simulink model "Noa_Nofusion"  (R2020b)
settings: Solver=FixedStepDiscrete  StartTime=0.0  StopTime=Inf  FixedStep=0.01  RelTol=1e-3
PostLoadFcn:
  | if any(exist('dsrtsu_mdlpostloadfcn', 'file') ~= 0), dsrtsu_mdlpostloadfcn('Execute', bdroot); end
InitFcn:
  | , if any(exist('rtifpga_mdlclblib', 'file') ~= 0), rtifpga_mdlclblib('Init', bdroot); end,
  | , if any(exist('dsmpb_private', 'file') ~= 0), dsmpb_private('dsmpb_mdlclblib', 'Init', bdroot); end,
undefined symbols (not defined in the file or in its folder): ACC_TimeGap_DecSetSwt, ACC_TimeGap_IncSetSwt, AccelPedalPosn, AccelPedalPosnVldty, AccelPedlPosnDiagc, AccPedalOverride, ACU_ShiftInProgress, ADAS_Posn_CurLane, AESSwtReq, ALC_SwtReq, BrkPedalSts, CC_ACC_CANCEL_OFFSwt, CC_ACC_CRUISE_OFFSwt, CC_ACC_DecSetSpd_SetSwt, CC_ACC_IncSetSpd_ResuSwt, CC_ACCSwtErr, CharSpd_ms, CSA_NODE, CURRENT_GEAR, CurrentGearValid, DiscIntNeverNeededParam, DrvDoorSts, DrvSBR, DrvTrqReqOvld, ECMACCInterface, ECMRespACC, ELKSwtReq, EngLimpHomeSts, EngSpd, EngState, EngState_PHEV, EngTrqMaxActSpd, EngTrqMinAct, EPS_DrvInpTrqVal_HighReslolution, EPS_FailSts, EPS_LKATorqOvrlDlvd, EPS_LKATorqOvrlDlvdVld, EPS_LKATrqOvlDlvdSts, EPS_SteerMod, EPS_TrqSnsrSts, EQ4_APPINFO, EQ4_LA_ELEM, EQ4_LA_HDR, EQ4_LAP_ELEM, EQ4_LAP_HDR, EQ4_LH_ELEM, EQ4_LH_HDR, EQ4_LRE_ELEM, EQ4_LRE_HDR, ESS_PedSwtReq, ESS_VehSwtReq, FFogLmpSts_F_Pbox, FLWheelDriveDirection, FLWheelSpd, FrntWiprSwtSts, FrntWshrSwtSts, FRWheelDriveDirection, FRWheelSpd, HazardLmpSwtSts, HCU_AccelPedalPosn_Diag ... (+151)
libraries: simulink x144, dsmpblib x33, canfdmsglib x10
(part 9 of 20)

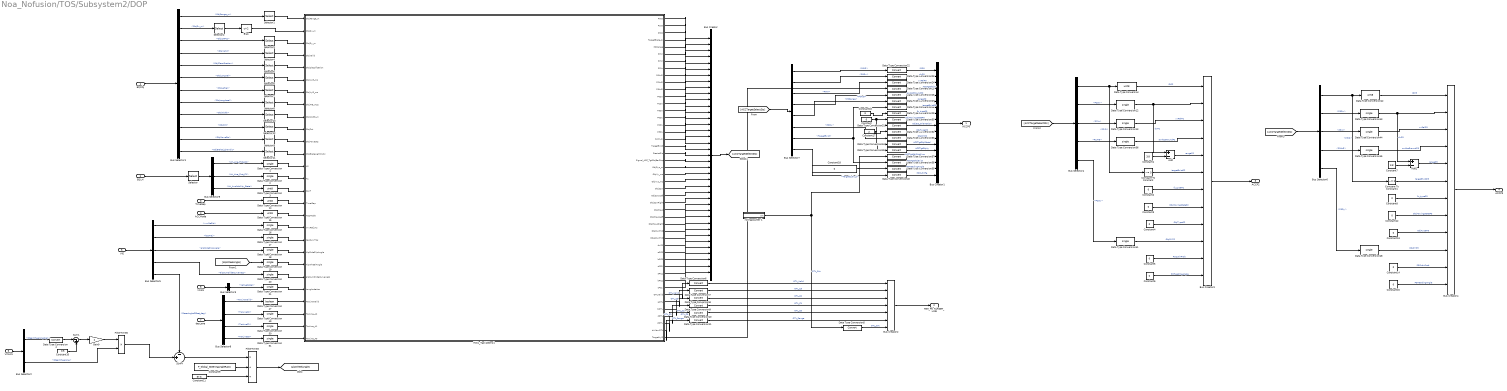
== system Noa_Nofusion/TOS/Subsystem2/DOP ==
  EQObj : Inport
  EQLH : Inport  Port=2
  TimeGap : Inport  Port=3
  ACCMode : Inport  Port=4
  VIE : Inport  Port=5
  VCAN : Inport  Port=6
  desLane : Inport  Port=7
  Add : Sum  Inputs=+-
  Add1 : Sum  Inputs=+-
  Bias : Bias  Bias=2
  Bus Creator : BusCreator  Inputs=39
  Bus Creator1 : BusCreator  Inputs=18  OutDataTypeStr=Bus: TOS_ACCP0_BUS  NonVirtualBus=on
  Bus Creator2 : BusCreator  Inputs=7  OutDataTypeStr=Bus: TOS_P0_TARGET_LINE_BUS  NonVirtualBus=on
  Bus Creator3 : BusCreator  Inputs=12  OutDataTypeStr=Bus: TOS_ACCP2_BUS  NonVirtualBus=on
  Bus Creator4 : BusCreator  Inputs=12  OutDataTypeStr=Bus: TOS_ACCP3_BUS  NonVirtualBus=on
  Bus Selector4 : BusSelector  OutputSignals=P2ID,P2Dx,P2Vr,P2ArG,P2Dy
  Bus Selector6 : BusSelector  OutputSignals=P3ID,P3Dx,P3Vr,P3ArG,P3Dy
  Bus Selector7 : BusSelector  OutputSignals=P0ID,P0Dx,P0Vr,P0ArG,P0Range,P0Dy,TargetExist,TargetCutIn_b
  Bus Selector9 : BusSelector  OutputSignals=LH_Line_First_C2,LH_Line_First_C1,LH_Availability_State
  Bus Selector1 : BusSelector  OutputSignals=ObjRange_m,ObjDx_m,ObjLatPos,ObjValid,ObjClassification,ObjLongVel,ObjLatVel,ObjLongAccel,ObjWidth,ObjCnt,ObjMoveSts,ObjBrakeLightIndic
  Bus Selector2 : BusSelector  OutputSignals=CSA_NODE.CSA2_MSG.SteerWheelAngSign,CSA_NODE.CSA2_MSG.SteerWheelAng
  Bus Selector3 : BusSelector  OutputSignals=ABM_NODE.ABM2_MSG.VehLgtAccel
  Bus Selector5 : BusSelector  OutputSignals=vxvRefMs,kapTraj,alpSideSlipAngle,alpSumSlideCurveness,SteerAngleOffset_deg
  Bus Selector8 : BusSelector  OutputSignals=TarLineValid,TarLineC2,TarLineC1,TarLineC0
  Compare To Constant : simulink/Logic and Bit Operations/Compare To Constant  relop=~=  const=0  OutDataTypeStr=boolean
  Compare To Constant1 : simulink/Logic and Bit Operations/Compare To Constant  relop=~=  const=0  OutDataTypeStr=boolean
  Constant : Constant  Value=0
  Constant1 : Constant  Value=3.8  OutDataTypeStr=single
  Constant10 : Constant  Value=0.5  OutDataTypeStr=single
  Constant11 : Constant  Value=57.3  OutDataTypeStr=single
  Constant{2..4,8,12..13} (6 alike) : Constant  Value=0  OutDataTypeStr=uint8
  Constant{5..6,14..15} (4 alike) : Constant  Value=0  OutDataTypeStr=single
  Constant16 : Constant  Value=3
  Constant17 : Constant  Value=2
  Constant18 : Constant  Value=0
  Constant7 : Constant  Value=3.8  OutDataTypeStr=single
  Constant9 : Constant  Value=P_Global_SteeringAngleRatio
  Data Type Conversion{,3,14..15,42} (5 alike) : DataTypeConversion  OutDataTypeStr=uint8
  Data Type Conversion{1..2,12..13,16..21,36,41,43..45,48..51} (19 alike) : DataTypeConversion  OutDataTypeStr=single
  Data Type Conversion{4..11,22..35,37..40} (26 alike) : DataTypeConversion
  Data Type Conversion47 : DataTypeConversion  OutDataTypeStr=boolean
  FilterTime3 : Product  Inputs=*//  RndMeth=Zero
  FilterTime6 : Product  Inputs=**  RndMeth=Zero
  Gain9 : Gain  Gain=2
  HWA_Task100ms1 : Subsystem
  Selector : Selector  InputPortWidth=2  IndexOptions=Index vector (dialog)  Indices=1  OutputSizes=1
  Selector{1..12} (12 alike) : Selector  InputPortWidth=20  IndexOptions=Index vector (dialog)  Indices=[1:15]  OutputSizes=1
  Sum1 : Sum  Inputs=|-+
  Sum4 : Sum  Inputs=-+|
  VCAN1 : InportShadow  Port=6
  rollingcounter 1 : Subsystem
  ACCP0 : Outport  OutDataTypeStr=Bus: TOS_ACCP0_BUS
  TEM_P0_TARGET_LINE : Outport  Port=2  OutDataTypeStr=Bus: TOS_P0_TARGET_LINE_BUS  PortDimensions=1  BusOutputAsStruct=on
  ACCP2 : Outport  Port=3  OutDataTypeStr=Bus: TOS_ACCP2_BUS
  ACCP3 : Outport  Port=4  OutDataTypeStr=Bus: TOS_ACCP3_BUS
  wires:
  EQLH/1 -> Selector/1
  EQObj/1 -> Bus Selector1/1
  Bus Selector8/4 -> Data Type Conversion51/1  "<TarLineC0>"
  Data Type Conversion51/1 -> HWA_Task100ms1/27(TarLine_A0)
  Constant18/1 -> Data Type Conversion39/1
  HWA_Task100ms1/46(TargetVyG) -> Data Type Conversion25/1
  Constant17/1 -> Data Type Conversion32/1
  Constant16/1 -> Data Type Conversion29/1
  Selector2/1 -> Bias/1
  [ACCTargetSelectSts] -> Bus Selector6/1
  Bus Selector6/1 -> Compare To Constant1/1, Data Type Conversion42/1  "<P3ID>"
  Data Type Conversion42/1 -> Bus Creator4/1  "IDP3"
  Bus Selector6/2 -> Data Type Conversion43/1  "<P3Dx>"
  Data Type Conversion43/1 -> Add1/1, Bus Creator4/2  "dxP3"
  Bus Selector6/3 -> Data Type Conversion44/1  "<P3Vr>"
  Data Type Conversion44/1 -> Bus Creator4/3  "vxRelP3"
  Bus Selector6/4 -> Data Type Conversion45/1  "<P3ArG>"
  Data Type Conversion45/1 -> Bus Creator4/4  "axAbsGroundP3"
  Add1/1 -> Bus Creator4/5  "rangeP3"
  Constant7/1 -> Add1/2
  Compare To Constant1/1 -> Bus Creator4/6  "targetExistP3"
  Constant8/1 -> Bus Creator4/7  "fu_typeP3"
  Constant12/1 -> Bus Creator4/8  "ObjMovingStateP3"
  Constant13/1 -> Bus Creator4/9  "ObjTypeP3"
  Bus Selector6/5 -> Data Type Conversion48/1  "<P3Dy>"
  Data Type Conversion48/1 -> Bus Creator4/10  "ObjDYP3"
  Constant14/1 -> Bus Creator4/11  "P3CutinProb"
  Constant15/1 -> Bus Creator4/12  "P3HeadingAngle"
  Bus Creator4/1 -> ACCP3/1
  Bus Creator3/1 -> ACCP2/1
  Constant6/1 -> Bus Creator3/12  "P2HeadingAngle"
  Constant5/1 -> Bus Creator3/11  "P2CutinProb"
  Data Type Conversion41/1 -> Bus Creator3/10  "ObjDYP2"
  Bus Selector4/5 -> Data Type Conversion41/1  "<P2Dy>"
  Constant4/1 -> Bus Creator3/9  "ObjTypeP2"
  Constant3/1 -> Bus Creator3/8  "ObjMovingStateP2"
  Constant2/1 -> Bus Creator3/7  "fu_typeP2"
  Compare To Constant/1 -> Bus Creator3/6  "targetExistP2"
  Constant1/1 -> Add/2
  Add/1 -> Bus Creator3/5  "rangeP2"
  Data Type Conversion36/1 -> Bus Creator3/4  "axAbsGroundP2"
  Bus Selector4/4 -> Data Type Conversion36/1  "<P2ArG>"
  Data Type Conversion13/1 -> Bus Creator3/3  "vxRelP2"
  Bus Selector4/3 -> Data Type Conversion13/1  "<P2Vr>"
  Data Type Conversion12/1 -> Bus Creator3/2, Add/1  "dxP2"
  Bus Selector4/2 -> Data Type Conversion12/1  "<P2Dx>"
  Data Type Conversion/1 -> Bus Creator3/1  "IDP2"
  Bus Selector4/1 -> Data Type Conversion/1, Compare To Constant/1  "<P2ID>"
  [ACCTargetSelectSts] -> Bus Selector4/1
  Selector12/1 -> HWA_Task100ms1/10(ObjCnt)
  Selector11/1 -> HWA_Task100ms1/12(ObjBrakeLightIndic)
  Selector10/1 -> HWA_Task100ms1/9(ObjWidth_m)
  Selector9/1 -> HWA_Task100ms1/11(ObjMoveSts)
  Selector8/1 -> HWA_Task100ms1/8(ObjArG_ms2)
  Selector7/1 -> HWA_Task100ms1/7(ObjVyG_ms)
  Selector6/1 -> HWA_Task100ms1/6(ObjVxG_ms)
  Selector5/1 -> HWA_Task100ms1/5(ObjClassification)
  Selector4/1 -> HWA_Task100ms1/4(ObjValid)
  Selector3/1 -> HWA_Task100ms1/3(ObjDy_m)
  Bias/1 -> HWA_Task100ms1/2(ObjDx_m)
  Selector1/1 -> HWA_Task100ms1/1(ObjRange_m)
  Selector/1 -> Bus Selector9/1
  Data Type Conversion11/1 -> Bus Creator2/6  "OTL_Range"
  Data Type Conversion10/1 -> Bus Creator2/5  "OTL_C0"
  Data Type Conversion9/1 -> Bus Creator2/4  "OTL_C1"
  Data Type Conversion8/1 -> Bus Creator2/3  "OTL_C2"
  Data Type Conversion7/1 -> Bus Creator2/2  "OTL_C3"
  Data Type Conversion6/1 -> Bus Creator2/1  "OTL_Valid"
  Data Type Conversion5/1 -> Bus Creator2/7  "OTL_Cnt"
  Bus Creator2/1 -> TEM_P0_TARGET_LINE/1
  HWA_Task100ms1/42(bOTL) -> Data Type Conversion8/1  "OTL_C2"
  HWA_Task100ms1/41(aOTL) -> Data Type Conversion7/1  "OTL_C3"
  HWA_Task100ms1/40(OTLValid) -> Data Type Conversion6/1  "OTL_Valid"
  HWA_Task100ms1/43(cOTL) -> Data Type Conversion9/1  "OTL_C1"
  rollingcounter 1/1(cnt) -> Data Type Conversion5/1, Data Type Conversion37/1  "OTL_Cnt"
  HWA_Task100ms1/45(dxMaxOTL) -> Data Type Conversion11/1  "OTL_Range"
  HWA_Task100ms1/44(dOTL) -> Data Type Conversion10/1  "OTL_C0"
  Data Type Conversion4/1 -> Sum1/1
  Bus Selector2/2 -> FilterTime6/2  "<SteerWheelAng>"
  Bus Selector2/1 -> Data Type Conversion4/1  "<SteerWheelAngSign>"
  Sum1/1 -> Gain9/1
  Gain9/1 -> FilterTime6/1
  Constant10/1 -> Sum1/2
  VCAN1/1 -> Bus Selector2/1
  Constant9/1 -> FilterTime3/2
  Bus Selector5/5 -> Sum4/1  "<SteerAngleOffset_deg>"
  FilterTime3/1 -> [alpWheelAngle]
  Sum4/1 -> FilterTime3/1
  Constant11/1 -> FilterTime3/3
  FilterTime6/1 -> Sum4/2
  HWA_Task100ms1/34(aPC0) -> Bus Creator/34
  HWA_Task100ms1/38(bPC1) -> Bus Creator/38
  Bus Selector7/1 -> Data Type Conversion22/1  "<P0ID>"
  Data Type Conversion3/1 -> HWA_Task100ms1/15(Conf)
  Data Type Conversion22/1 -> Bus Creator1/1  "IDP0"
  Data Type Conversion27/1 -> Bus Creator1/6  "rangeP0"
  Data Type Conversion1/1 -> HWA_Task100ms1/13(A2)
  HWA_Task100ms1/2(P2ID) -> Bus Creator/2
  Data Type Conversion2/1 -> HWA_Task100ms1/14(A1)
  Data Type Conversion37/1 -> Bus Creator1/15  "ACCTgtObjCntAlive"
  HWA_Task100ms1/1(P0ID) -> Bus Creator/1
  Bus Selector3/1 -> Data Type Conversion21/1  "<VehLgtAccel>"
  Bus Selector1/9 -> Selector10/1  "<ObjWidth>"
  Data Type Conversion19/1 -> HWA_Task100ms1/21(AlpWheelAngle)
  Bus Selector7/3 -> Data Type Conversion24/1  "<P0Vr>"
  Bus Selector9/1 -> Data Type Conversion1/1  "<LH_Line_First_C2>"
  VIE/1 -> Bus Selector5/1
  Bus Creator1/1 -> ACCP0/1
  Data Type Conversion38/1 -> Bus Creator1/16  "ACCTgtObjExist"
  Bus Selector7/6 -> Data Type Conversion33/1  "<P0Dy>"
  Bus Selector7/2 -> Data Type Conversion23/1  "<P0Dx>"
  Data Type Conversion29/1 -> Bus Creator1/8  "fu_typeP0"
  Bus Selector7/8 -> Data Type Conversion40/1  "<TargetCutIn_b>"
  HWA_Task100ms1/32(ObjqDycHist) -> Bus Creator/32
  Data Type Conversion32/1 -> Bus Creator1/11  "ObjTypeP0"
  Data Type Conversion35/1 -> Bus Creator1/14  "ACCTgtObjAy"
  VCAN/1 -> Bus Selector3/1
  Data Type Conversion34/1 -> Bus Creator1/13  "ACCTgtObjObstcl"
  Bus Selector8/1 -> Data Type Conversion47/1  "<TarLineValid>"
  Bus Selector5/1 -> Data Type Conversion16/1  "<vxvRefMs>"
  Data Type Conversion17/1 -> HWA_Task100ms1/19(kapCurvTraj)
  Data Type Conversion28/1 -> Bus Creator1/7  "targetExistP0"
  Bus Selector1/7 -> Selector7/1  "<ObjLatVel>"
  HWA_Task100ms1/8(P3Vr) -> Bus Creator/8
  Bus Selector1/8 -> Selector8/1  "<ObjLongAccel>"
  Data Type Conversion49/1 -> HWA_Task100ms1/25(TarLine_A2)
  ACCMode/1 -> Data Type Conversion15/1
  HWA_Task100ms1/22(ObjDyc_m) -> Bus Creator/22
  Data Type Conversion18/1 -> HWA_Task100ms1/20(AlpSideSlipAngle)
  Data Type Conversion30/1 -> Bus Creator1/9  "ObjMovingStateP0"
  HWA_Task100ms1/11(P3ArG) -> Bus Creator/11
  Data Type Conversion25/1 -> Bus Creator1/4  "ACCTgtObjVy"
  TimeGap/1 -> Data Type Conversion14/1
  Data Type Conversion23/1 -> Bus Creator1/2  "dxP0"
  Data Type Conversion21/1 -> HWA_Task100ms1/23(LongitudeAcc)
  Bus Creator/1 -> [ACCTargetSelectSts]
  HWA_Task100ms1/31(ObjDycHist) -> Bus Creator/31
  Bus Selector1/5 -> Selector5/1  "<ObjClassification>"
  Bus Selector7/5 -> Data Type Conversion27/1  "<P0Range>"
  Bus Selector5/2 -> Data Type Conversion17/1  "<kapTraj>"
  Bus Selector1/3 -> Selector3/1  "<ObjLatPos>"
  Constant/1 -> Data Type Conversion30/1, Data Type Conversion31/1, Data Type Conversion34/1, Data Type Conversion35/1
  Data Type Conversion47/1 -> HWA_Task100ms1/24(TarLineValid)
  HWA_Task100ms1/4(TargetBrake_b) -> Bus Creator/4
  Data Type Conversion14/1 -> HWA_Task100ms1/16(TimeGap)
  HWA_Task100ms1/15(P0Dy) -> Bus Creator/15
  HWA_Task100ms1/33(dxC0) -> Bus Creator/33
  Data Type Conversion39/1 -> Bus Creator1/17  "P0HeadingAngle"
  HWA_Task100ms1/21(Signal_ACC_TgtObjBarDisp) -> Bus Creator/21
  HWA_Task100ms1/24(ObjVyc_ms) -> Bus Creator/24
  HWA_Task100ms1/16(P2Dy) -> Bus Creator/16
  Bus Selector8/3 -> Data Type Conversion50/1  "<TarLineC1>"
  HWA_Task100ms1/30(ObjPlausRight) -> Bus Creator/30
  HWA_Task100ms1/13(P2Dx) -> Bus Creator/13
  Bus Selector1/11 -> Selector9/1  "<ObjMoveSts>"
  HWA_Task100ms1/35(bPC0) -> Bus Creator/35
  Data Type Conversion16/1 -> HWA_Task100ms1/18(VxvRef_ms)
  Bus Selector9/2 -> Data Type Conversion2/1  "<LH_Line_First_C1>"
  HWA_Task100ms1/18(CutIn_b) -> Bus Creator/18
  HWA_Task100ms1/27(ObjSpwRight) -> Bus Creator/27
  [ACCTargetSelectSts] -> Bus Selector7/1
  HWA_Task100ms1/3(P3ID) -> Bus Creator/3
  HWA_Task100ms1/20(DesireDis) -> Bus Creator/20
  Bus Selector7/4 -> Data Type Conversion26/1  "<P0ArG>"
  Data Type Conversion31/1 -> Bus Creator1/10  "Object_Orientation"
  Data Type Conversion50/1 -> HWA_Task100ms1/26(TarLine_A1)
  Bus Selector1/1 -> Selector1/1  "<ObjRange_m>"
  Bus Selector1/6 -> Selector6/1  "<ObjLongVel>"
  Bus Selector1/12 -> Selector11/1  "<ObjBrakeLightIndic>"
  Bus Selector5/3 -> Data Type Conversion18/1  "<alpSideSlipAngle>"
  HWA_Task100ms1/14(P3Dx) -> Bus Creator/14
  Data Type Conversion33/1 -> Bus Creator1/12  "ObjDYP0"
  Bus Selector5/4 -> Data Type Conversion20/1  "<alpSumSlideCurveness>"
  HWA_Task100ms1/9(P0ArG) -> Bus Creator/9
  HWA_Task100ms1/36(cPC0) -> Bus Creator/36
  HWA_Task100ms1/39(cPC1) -> Bus Creator/39
  HWA_Task100ms1/12(P0Dx) -> Bus Creator/12
  HWA_Task100ms1/17(P3Dy) -> Bus Creator/17
  HWA_Task100ms1/19(TargetExist) -> Bus Creator/19
  Bus Selector1/10 -> Selector12/1  "<ObjCnt>"
  HWA_Task100ms1/10(P2ArG) -> Bus Creator/10
  HWA_Task100ms1/26(ObjSpwLeft) -> Bus Creator/26
  HWA_Task100ms1/37(aPC1) -> Bus Creator/37
  HWA_Task100ms1/5(P0Range) -> Bus Creator/5
  Data Type Conversion26/1 -> Bus Creator1/5  "axAbsGroundP0"
  Bus Selector1/2 -> Selector2/1  "<ObjDx_m>"
  HWA_Task100ms1/28(ObjPlaus) -> Bus Creator/28
  Data Type Conversion24/1 -> Bus Creator1/3  "vxRelP0"
  Bus Selector8/2 -> Data Type Conversion49/1  "<TarLineC2>"
  Bus Selector1/4 -> Selector4/1  "<ObjValid>"
  HWA_Task100ms1/7(P2Vr) -> Bus Creator/7
  HWA_Task100ms1/29(ObjPlausLeft) -> Bus Creator/29
  Data Type Conversion40/1 -> Bus Creator1/18  "P0CutInflg"
  desLane/1 -> Bus Selector8/1
  Bus Selector9/3 -> Data Type Conversion3/1  "<LH_Availability_State>"
  [alpWheelAngle] -> Data Type Conversion19/1
  HWA_Task100ms1/25(ObjSpw) -> Bus Creator/25
  HWA_Task100ms1/6(P0Vr) -> Bus Creator/6
  Bus Selector7/7 -> Data Type Conversion38/1, Data Type Conversion28/1  "<TargetExist>"
  Data Type Conversion15/1 -> HWA_Task100ms1/17(ACCMode)
  HWA_Task100ms1/23(ObjVy_ms) -> Bus Creator/23
  Data Type Conversion20/1 -> HWA_Task100ms1/22(alpSumSlideCurveness)

== system Noa_Nofusion/TOS/Subsystem2/ObjMatrixTransit ==
  EQ4_OBJ : Inport
  Bus Creator : BusCreator  Inputs=14
  Bus Selector4 : BusSelector  OutputSignals=EQ4_OBJ_HDR.OBJ_Sync_ID,EQ4_OBJ_HDR.OBJ_VRU_Count,EQ4_OBJ_HDR.OBJ_VD_Count,EQ4_OBJ_HDR.OBJ_General_OBJ_Count,EQ4_OBJ_HDR.OBJ_Animal_Count,EQ4_OBJ_ELEM
  Data Type Conversion : DataTypeConversion
  IFV2FrontBumper : Constant  Value=1.7  OutDataTypeStr=single
  IFV2RearAxis : Constant  Value=2.1  OutDataTypeStr=single
  Subsystem : Subsystem
  Sum : Sum  Inputs=++++
  Sum1 : Sum  Inputs=|-+
  Sum5 : Sum  Inputs=++|
  Terminator1 : Terminator
  VisObj : Outport
  wires:
  Subsystem/13(P) -> Terminator1/1
  EQ4_OBJ/1 -> Bus Selector4/1
  Bus Selector4/5 -> Sum/4  "<OBJ_Animal_Count>"
  Bus Selector4/1 -> Data Type Conversion/1  "<OBJ_Sync_ID>"
  Bus Selector4/2 -> Sum/1  "<OBJ_VRU_Count>"
  Bus Selector4/3 -> Sum/2  "<OBJ_VD_Count>"
  Bus Selector4/4 -> Sum/3  "<OBJ_General_OBJ_Count>"
  Sum/1 -> Subsystem/1(Count)
  Bus Selector4/6 -> Subsystem/2(<EQ4_OBJ_ELEM>)  "<EQ4_OBJ_ELEM>"
  Subsystem/1(ObjID) -> Bus Creator/2  "ObjID"
  Bus Creator/1 -> VisObj/1  "ObjSts"
  IFV2FrontBumper/1 -> Sum1/1
  Data Type Conversion/1 -> Bus Creator/1  "Cnt"
  IFV2RearAxis/1 -> Sum5/2
  Sum5/1 -> Bus Creator/14  "ObjDx_m"
  Subsystem/11(ObjMoveSts) -> Bus Creator/12  "ObjMoveSts"
  Sum1/1 -> Bus Creator/13  "ObjRange_m"
  Subsystem/10(ObjCnt) -> Bus Creator/11  "ObjCnt"
  Subsystem/8(ObjLongVel) -> Bus Creator/9  "ObjLongVel"
  Subsystem/12(ObjLongPos) -> Sum1/2, Sum5/1
  Subsystem/9(ObjWidth) -> Bus Creator/10  "ObjWidth"
  Subsystem/3(ObjBrakeLightIndic) -> Bus Creator/4  "ObjBrakeLightIndic"
  Subsystem/5(ObjLatPos) -> Bus Creator/6  "ObjLatPos"
  Subsystem/7(ObjLongAccel) -> Bus Creator/8  "ObjLongAccel"
  Subsystem/2(ObjValid) -> Bus Creator/3  "ObjValid"
  Subsystem/4(ObjClassification) -> Bus Creator/5  "ObjClassification"
  Subsystem/6(ObjLatVel) -> Bus Creator/7  "ObjLatVel"

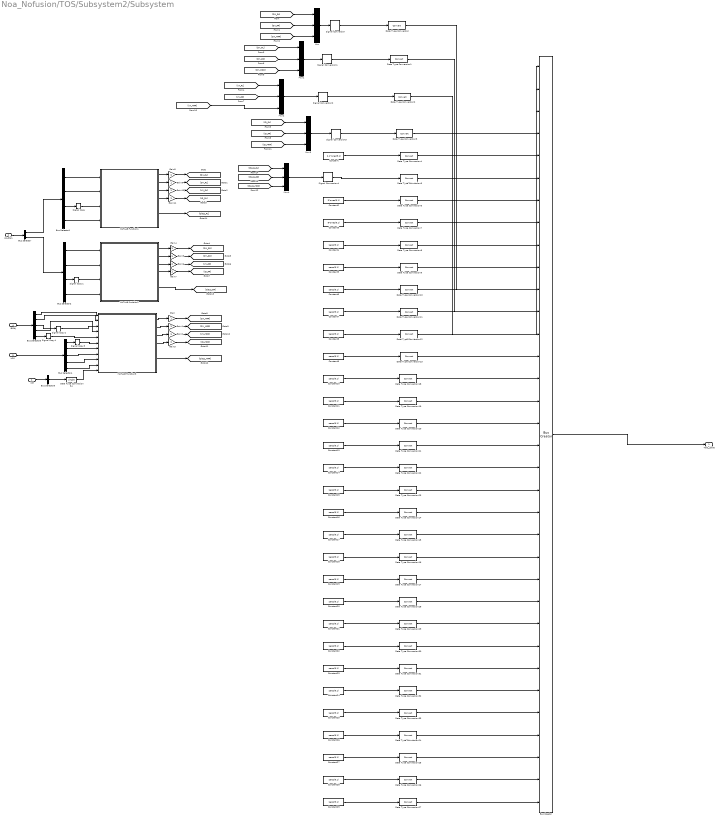
== system Noa_Nofusion/TOS/Subsystem2/Subsystem ==
  VIE : Inport
  LC_Obj1 : Inport  Port=2
  LSM : Inport  Port=3
  IEObj : Inport  Port=4
  Bus Creator : BusCreator  Inputs=34  OutDataTypeStr=Bus: TOS_LCKIE_BUS  NonVirtualBus=on
  Bus Selector : BusSelector  OutputSignals=RL,RR
  Bus Selector1 : BusSelector  OutputSignals=ObjID,ObjDy,ObjDx,ObjVx
  Bus Selector2 : BusSelector  OutputSignals=ObjID,ObjDy,ObjDx,ObjVx
  Bus Selector3 : BusSelector  OutputSignals=ObjID,ObjLatPos,ObjDx_m,ObjLongVel,ObjClass
  Bus Selector4 : BusSelector  OutputSignals=LSM_LCK.LCKLineValid,LSM_LCK.LCKLineC0,LSM_LCK.LCKLineC1,LSM_LCK.LCKLineC2,LSM_LCK.LCKLineC3
  Bus Selector5 : BusSelector  OutputSignals=vxvRefMs
  Constant : Constant  Value=2.1*ones(9,1)  OutDataTypeStr=single
  Constant{4..29} (26 alike) : Constant  Value=zeros(9,1)  OutDataTypeStr=single
  Constant2 : Constant  Value=3*ones(9,1)  OutDataTypeStr=uint8
  Constant3 : Constant  Value=8*ones(9,1)  OutDataTypeStr=single
  Data Type Conversion{,1..33} (34 alike) : DataTypeConversion
  Data Type Conversion34 : DataTypeConversion  OutDataTypeStr=single
  Gain{,1..11} (12 alike) : Gain
  MATLAB Function1 : MATLAB Function  TreatAsAtomicUnit=on
  MATLAB Function2 : MATLAB Function  TreatAsAtomicUnit=on
  MATLAB Function3 : MATLAB Function  TreatAsAtomicUnit=on
  Mux{,1..4} (5 alike) : Mux  Inputs=3
  Signal Conversion{,1..4} (5 alike) : SignalConversion  OverrideOpt=off
  Signal Copy{,1..4} (5 alike) : SignalConversion  OverrideOpt=off
  TOS_LCKIE : Outport  OutDataTypeStr=Bus: TOS_LCKIE_BUS
  wires:
  Bus Selector2/2 -> MATLAB Function2/2(ObjDy)  "<ObjDy>"
  Bus Selector/2 -> Bus Selector2/1  "<RR>"
  LC_Obj1/1 -> Bus Selector/1
  Bus Selector1/3 -> Signal Copy/1  "<ObjDx>"
  Bus Selector1/2 -> MATLAB Function1/2(ObjDy)  "<ObjDy>"
  Bus Selector1/4 -> MATLAB Function1/4(ObjVx)  "<ObjVx>"
  Bus Selector4/3 -> MATLAB Function3/8(C1)  "<LCKLineC1>"
  Bus Selector2/1 -> MATLAB Function2/1(ObjID)  "<ObjID>"
  Bus Selector1/1 -> MATLAB Function1/1(ObjID)  "<ObjID>"
  Bus Selector2/3 -> Signal Copy1/1  "<ObjDx>"
  Bus Selector2/4 -> MATLAB Function2/4(ObjVx)  "<ObjVx>"
  Bus Selector3/4 -> MATLAB Function3/4(ObjVx)  "<ObjLongVel>"
  Bus Selector3/3 -> Signal Copy2/1  "<ObjDx_m>"
  Bus Selector4/2 -> MATLAB Function3/7(C0)  "<LCKLineC0>"
  Bus Selector3/2 -> MATLAB Function3/2(ObjDy)  "<ObjLatPos>"
  Bus Selector3/1 -> MATLAB Function3/1(ObjID)  "<ObjID>"
  LSM/1 -> Bus Selector4/1
  Bus Selector/1 -> Bus Selector1/1  "<RL>"
  Bus Selector4/1 -> Signal Copy3/1  "<LCKLineValid>"
  Bus Selector4/5 -> MATLAB Function3/10(C3)  "<LCKLineC3>"
  Bus Selector4/4 -> MATLAB Function3/9(C2)  "<LCKLineC2>"
  IEObj/1 -> Bus Selector3/1
  MATLAB Function1/1(Dx) -> Gain8/1
  MATLAB Function1/2(Dy) -> Gain9/1
  MATLAB Function1/3(Vx) -> Gain10/1
  MATLAB Function1/4(ID) -> Gain11/1
  MATLAB Function2/1(Dx) -> Gain4/1
  MATLAB Function2/2(Dy) -> Gain5/1
  MATLAB Function2/3(Vx) -> Gain6/1
  MATLAB Function2/4(ID) -> Gain7/1
  MATLAB Function3/1(Dx) -> Gain/1
  MATLAB Function3/2(Dy) -> Gain1/1
  MATLAB Function3/3(Vx) -> Gain2/1
  MATLAB Function3/4(ID) -> Gain3/1
  [DX_RL] -> Mux/1
  [DX_RR] -> Mux/2
  [DX_MRR] -> Mux/3
  [DY_RR] -> Mux1/2
  [DY_RL] -> Mux1/1
  [DY_MRR] -> Mux1/3
  [VX_RL] -> Mux2/1
  [VX_RR] -> Mux2/2
  [ID_RL] -> Mux3/1
  [ID_RR] -> Mux3/2
  [ID_MRR] -> Mux3/3
  Mux/1 -> Signal Conversion/1
  Mux1/1 -> Signal Conversion1/1
  Mux2/1 -> Signal Conversion2/1
  Mux3/1 -> Signal Conversion3/1
  Constant/1 -> Data Type Conversion4/1  "Object_Width"
  Mux4/1 -> Signal Conversion4/1  "Object_Type"
  Constant2/1 -> Data Type Conversion6/1  "Object_Fus_Type"
  Bus Creator/1 -> TOS_LCKIE/1
  Constant3/1 -> Data Type Conversion7/1  "Object_Length"
  Constant4/1 -> Data Type Conversion8/1  "Object_Hight"
  Constant5/1 -> Data Type Conversion9/1  "Object_HeadingAngle"
  Constant6/1 -> Data Type Conversion10/1  "Object_YawAngle"
  Constant7/1 -> Data Type Conversion11/1  "Object_MovingState"
  Constant8/1 -> Data Type Conversion12/1  "Object_Orientation"
  Constant9/1 -> Data Type Conversion13/1  "Object_VY"
  Constant10/1 -> Data Type Conversion18/1  "Object_Std_AX"
  Constant11/1 -> Data Type Conversion19/1  "Object_Std_AY"
  Constant12/1 -> Data Type Conversion20/1  "Object_Std_DX"
  Constant13/1 -> Data Type Conversion21/1  "Object_Std_DY"
  Constant14/1 -> Data Type Conversion22/1  "Object_Std_VX"
  Constant15/1 -> Data Type Conversion23/1  "Object_Std_VY"
  Constant16/1 -> Data Type Conversion14/1  "Object_AX"
  Constant17/1 -> Data Type Conversion15/1  "Object_AY"
  Constant18/1 -> Data Type Conversion16/1  "Object_Std_Length"
  Constant19/1 -> Data Type Conversion17/1  "Object_Std_Width"
  Constant20/1 -> Data Type Conversion28/1  "Object_Std_HeadingAngle"
  Constant21/1 -> Data Type Conversion29/1  "Object_Type_Prob"
  Constant22/1 -> Data Type Conversion30/1  "Object_ExistProb"
  Constant23/1 -> Data Type Conversion31/1  "Object_ObstacleProb"
  Constant24/1 -> Data Type Conversion32/1  "Object_Age"
  Constant25/1 -> Data Type Conversion33/1  "cutIn"
  Constant26/1 -> Data Type Conversion24/1  "CurrentLane_Prob"
  Constant27/1 -> Data Type Conversion25/1  "LeftLane_Prob"
  Constant28/1 -> Data Type Conversion26/1  "RightLane_Prob"
  Constant29/1 -> Data Type Conversion27/1  "ObjectIn_Lane"
  Data Type Conversion/1 -> Bus Creator/11  "Object_DX"
  Data Type Conversion1/1 -> Bus Creator/12  "Object_DY"
  Data Type Conversion2/1 -> Bus Creator/13  "Object_VX"
  Data Type Conversion3/1 -> Bus Creator/2  "Object_ID"
  Data Type Conversion4/1 -> Bus Creator/5  "Object_Width"
  Data Type Conversion5/1 -> Bus Creator/3  "Object_Type"
  Data Type Conversion6/1 -> Bus Creator/1  "Object_Fus_Type"
  Data Type Conversion7/1 -> Bus Creator/4  "Object_Length"
  Data Type Conversion8/1 -> Bus Creator/6  "Object_Hight"
  Data Type Conversion11/1 -> Bus Creator/9  "Object_MovingState"
  Data Type Conversion9/1 -> Bus Creator/7  "Object_HeadingAngle"
  Data Type Conversion10/1 -> Bus Creator/8  "Object_YawAngle"
  Data Type Conversion12/1 -> Bus Creator/10  "Object_Orientation"
  Data Type Conversion13/1 -> Bus Creator/14  "Object_VY"
  Data Type Conversion15/1 -> Bus Creator/22  "Object_AY"
  Data Type Conversion17/1 -> Bus Creator/24  "Object_Std_Width"
  Data Type Conversion18/1 -> Bus Creator/15  "Object_Std_AX"
  Data Type Conversion20/1 -> Bus Creator/17  "Object_Std_DX"
  Data Type Conversion19/1 -> Bus Creator/16  "Object_Std_AY"
  Data Type Conversion22/1 -> Bus Creator/19  "Object_Std_VX"
  Data Type Conversion21/1 -> Bus Creator/18  "Object_Std_DY"
  Data Type Conversion23/1 -> Bus Creator/20  "Object_Std_VY"
  Data Type Conversion24/1 -> Bus Creator/31  "CurrentLane_Prob"
  Data Type Conversion26/1 -> Bus Creator/33  "RightLane_Prob"
  Data Type Conversion25/1 -> Bus Creator/32  "LeftLane_Prob"
  Data Type Conversion29/1 -> Bus Creator/26  "Object_Type_Prob"
  Data Type Conversion30/1 -> Bus Creator/27  "Object_ExistProb"
  Data Type Conversion33/1 -> Bus Creator/30  "cutIn"
  Data Type Conversion32/1 -> Bus Creator/29  "Object_Age"
  Data Type Conversion31/1 -> Bus Creator/28  "Object_ObstacleProb"
  Data Type Conversion28/1 -> Bus Creator/25  "Object_Std_HeadingAngle"
  Data Type Conversion27/1 -> Bus Creator/34  "ObjectIn_Lane"
  Data Type Conversion14/1 -> Bus Creator/21  "Object_AX"
  Data Type Conversion16/1 -> Bus Creator/23  "Object_Std_Length"
  Signal Copy/1 -> MATLAB Function1/3(ObjDx)
  Signal Copy1/1 -> MATLAB Function2/3(ObjDx)
  Signal Copy2/1 -> MATLAB Function3/3(ObjDx)  "EQ4_DX"
  Signal Copy3/1 -> MATLAB Function3/6(L_Valid)
  Signal Conversion/1 -> Data Type Conversion/1  "LCKIE_DX"
  Signal Conversion1/1 -> Data Type Conversion1/1  "LCKIE_DY"
  Signal Conversion2/1 -> Data Type Conversion2/1  "LCKIE_VX"
  Signal Conversion3/1 -> Data Type Conversion3/1  "LCKIE_ID"
  Gain/1 -> [DX_MRR]
  Gain1/1 -> [DY_MRR]
  Gain2/1 -> [VX_MRR]
  Gain3/1 -> [ID_MRR]
  Gain4/1 -> [DX_RR]
  Gain6/1 -> [VX_RR]
  Gain5/1 -> [DY_RR]
  Gain7/1 -> [ID_RR]
  Gain10/1 -> [VX_RL]
  Gain8/1 -> [DX_RL]
  Gain9/1 -> [DY_RL]
  Gain11/1 -> [ID_RL]
  VIE/1 -> Bus Selector5/1
  Bus Selector5/1 -> Data Type Conversion34/1  "<vxvRefMs>"
  [VX_MRR] -> Mux2/3
  Data Type Conversion34/1 -> MATLAB Function3/11(vxv)
  MATLAB Function3/6(Class) -> [Class_MRR]
  MATLAB Function2/6(Class) -> [Class_RR]
  MATLAB Function1/6(Class) -> [Class_RL]
  [Class_RL] -> Mux4/1
  [Class_RR] -> Mux4/2
  [Class_MRR] -> Mux4/3
  Signal Conversion4/1 -> Data Type Conversion5/1  "Object_Type"
  Bus Selector3/5 -> Signal Copy4/1  "<ObjClass>"
  Signal Copy4/1 -> MATLAB Function3/5(ObjClass)  "EQ4_Type"

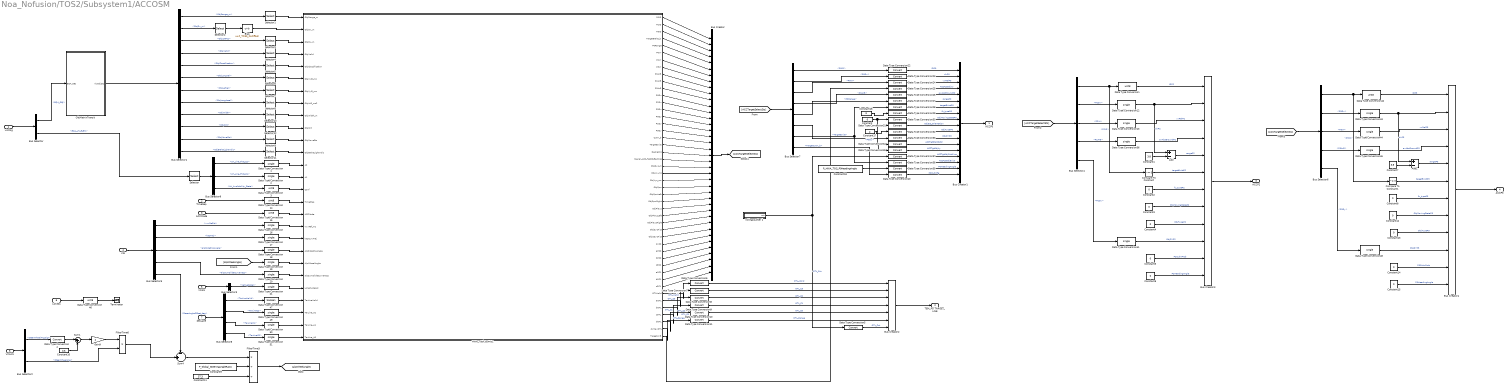
== system Noa_Nofusion/TOS2/Subsystem1/ACCOSM ==
  visMsg : Inport
  TimeGap : Inport  Port=2
  ACCMode : Inport  Port=3
  VIE : Inport  Port=4
  VCAN : Inport  Port=5
  LCKSts : Inport  Port=6
  desLane : Inport  Port=7
  Add : Sum  Inputs=+-
  Add1 : Sum  Inputs=+-
  Bias : Bias  Bias=P_TOSS_DxOffset
  Bus Creator : BusCreator  Inputs=39
  Bus Creator1 : BusCreator  Inputs=18  OutDataTypeStr=Bus: TOS_ACCP0_BUS  NonVirtualBus=on
  Bus Creator2 : BusCreator  Inputs=7  OutDataTypeStr=Bus: TOS_P0_TARGET_LINE_BUS  NonVirtualBus=on
  Bus Creator3 : BusCreator  Inputs=12  OutDataTypeStr=Bus: TOS_ACCP2_BUS  NonVirtualBus=on
  Bus Creator4 : BusCreator  Inputs=12  OutDataTypeStr=Bus: TOS_ACCP3_BUS  NonVirtualBus=on
  Bus Selector : BusSelector  OutputSignals=EQ4_OBJ,EQ4_LH.EQ4_LH_ELEM
  Bus Selector4 : BusSelector  OutputSignals=P2ID,P2Dx,P2Vr,P2ArG,P2Dy
  Bus Selector6 : BusSelector  OutputSignals=P3ID,P3Dx,P3Vr,P3ArG,P3Dy
  Bus Selector7 : BusSelector  OutputSignals=P0ID,P0Dx,P0Vr,P0ArG,P0Range,P0Dy,TargetExist,TargetCutIn_b
  Bus Selector9 : BusSelector  OutputSignals=LH_Line_First_C2,LH_Line_First_C1,LH_Availability_State
  Bus Selector1 : BusSelector  OutputSignals=ObjRange_m,ObjDx_m,ObjLatPos,ObjValid,ObjClassification,ObjLongVel,ObjLatVel,ObjLongAccel,ObjWidth,ObjCnt,ObjMoveSts,ObjBrakeLightIndic
  Bus Selector2 : BusSelector  OutputSignals=CSA_NODE.CSA2_MSG.SteerWheelAngSign,CSA_NODE.CSA2_MSG.SteerWheelAng
  Bus Selector3 : BusSelector  OutputSignals=ABM_NODE.ABM2_MSG.VehLgtAccel
  Bus Selector5 : BusSelector  OutputSignals=vxvRefMs,kapTraj,alpSideSlipAngle,alpSumSlideCurveness,SteerAngleOffset_deg
  Bus Selector8 : BusSelector  OutputSignals=TarLineValid,TarLineC2,TarLineC1,TarLineC0
  Compare To Constant : simulink/Logic and Bit Operations/Compare To Constant  relop=~=  const=0  OutDataTypeStr=boolean
  Compare To Constant1 : simulink/Logic and Bit Operations/Compare To Constant  relop=~=  const=0  OutDataTypeStr=boolean
  Constant : Constant  Value=0
  Constant1 : Constant  Value=3.8  OutDataTypeStr=single
  Constant10 : Constant  Value=0.5  OutDataTypeStr=single
  Constant11 : Constant  Value=57.3  OutDataTypeStr=single
  Constant{2..4,8,12..13} (6 alike) : Constant  Value=0  OutDataTypeStr=uint8
  Constant{5..6,14..15} (4 alike) : Constant  Value=0  OutDataTypeStr=single
  Constant16 : Constant  Value=3
  Constant17 : Constant  Value=2
  Constant18 : Constant  Value=P_HWA_TOS_P0HeadingAngle
  Constant7 : Constant  Value=3.8  OutDataTypeStr=single
  Constant9 : Constant  Value=P_Global_SteeringAngleRatio
  Data Type Conversion{,3,14..15,42,46} (6 alike) : DataTypeConversion  OutDataTypeStr=uint8
  Data Type Conversion{1..2,12..13,16..21,36,41,43..45,48..51} (19 alike) : DataTypeConversion  OutDataTypeStr=single
  Data Type Conversion{4..11,22..35,37..40} (26 alike) : DataTypeConversion
  Data Type Conversion47 : DataTypeConversion  OutDataTypeStr=boolean
  FilterTime3 : Product  Inputs=*//  RndMeth=Zero
  FilterTime6 : Product  Inputs=**  RndMeth=Zero
  Gain9 : Gain  Gain=2
  HWA_Task100ms1 : Subsystem
  ObjMatrixTransit : Subsystem
  Selector : Selector  InputPortWidth=2  IndexOptions=Index vector (dialog)  Indices=1  OutputSizes=1
  Selector{1..12} (12 alike) : Selector  InputPortWidth=20  IndexOptions=Index vector (dialog)  Indices=[1:15]  OutputSizes=1
  Sum1 : Sum  Inputs=|-+
  Sum4 : Sum  Inputs=-+|
  Terminator : Terminator
  VCAN1 : InportShadow  Port=5
  rollingcounter 1 : Subsystem
  ACCP0 : Outport  OutDataTypeStr=Bus: TOS_ACCP0_BUS
  TEM_P0_TARGET_LINE : Outport  Port=2  OutDataTypeStr=Bus: TOS_P0_TARGET_LINE_BUS  PortDimensions=1  BusOutputAsStruct=on
  ACCP2 : Outport  Port=3  OutDataTypeStr=Bus: TOS_ACCP2_BUS
  ACCP3 : Outport  Port=4  OutDataTypeStr=Bus: TOS_ACCP3_BUS
  wires:
  Bus Creator1/1 -> ACCP0/1
  Bus Selector8/4 -> Data Type Conversion51/1  "<TarLineC0>"
  Data Type Conversion20/1 -> HWA_Task100ms1/22(alpSumSlideCurveness)
  HWA_Task100ms1/23(ObjVy_ms) -> Bus Creator/23
  Data Type Conversion15/1 -> HWA_Task100ms1/17(ACCMode)
  Bus Selector7/7 -> Data Type Conversion28/1, Data Type Conversion38/1  "<TargetExist>"
  HWA_Task100ms1/6(P0Vr) -> Bus Creator/6
  HWA_Task100ms1/25(ObjSpw) -> Bus Creator/25
  [alpWheelAngle] -> Data Type Conversion19/1
  Bus Selector9/3 -> Data Type Conversion3/1  "<LH_Availability_State>"
  desLane/1 -> Bus Selector8/1
  Data Type Conversion40/1 -> Bus Creator1/18  "P0CutInflg"
  HWA_Task100ms1/29(ObjPlausLeft) -> Bus Creator/29
  HWA_Task100ms1/7(P2Vr) -> Bus Creator/7
  Bus Selector1/4 -> Selector4/1  "<ObjValid>"
  Bus Selector8/2 -> Data Type Conversion49/1  "<TarLineC2>"
  Data Type Conversion24/1 -> Bus Creator1/3  "vxRelP0"
  LCKSts/1 -> Data Type Conversion46/1
  HWA_Task100ms1/28(ObjPlaus) -> Bus Creator/28
  Bus Selector1/2 -> Selector2/1  "<ObjDx_m>"
  Data Type Conversion26/1 -> Bus Creator1/5  "axAbsGroundP0"
  HWA_Task100ms1/5(P0Range) -> Bus Creator/5
  HWA_Task100ms1/37(aPC1) -> Bus Creator/37
  HWA_Task100ms1/26(ObjSpwLeft) -> Bus Creator/26
  HWA_Task100ms1/10(P2ArG) -> Bus Creator/10
  Bus Selector1/10 -> Selector12/1  "<ObjCnt>"
  HWA_Task100ms1/19(TargetExist) -> Bus Creator/19
  HWA_Task100ms1/17(P3Dy) -> Bus Creator/17
  HWA_Task100ms1/12(P0Dx) -> Bus Creator/12
  HWA_Task100ms1/39(cPC1) -> Bus Creator/39
  HWA_Task100ms1/36(cPC0) -> Bus Creator/36
  HWA_Task100ms1/9(P0ArG) -> Bus Creator/9
  Bus Selector5/4 -> Data Type Conversion20/1  "<alpSumSlideCurveness>"
  Data Type Conversion33/1 -> Bus Creator1/12  "ObjDYP0"
  HWA_Task100ms1/14(P3Dx) -> Bus Creator/14
  Bus Selector5/3 -> Data Type Conversion18/1  "<alpSideSlipAngle>"
  Bus Selector1/12 -> Selector11/1  "<ObjBrakeLightIndic>"
  Bus Selector1/6 -> Selector6/1  "<ObjLongVel>"
  Bus Selector1/1 -> Selector1/1  "<ObjRange_m>"
  Data Type Conversion50/1 -> HWA_Task100ms1/26(TarLine_A1)
  Data Type Conversion31/1 -> Bus Creator1/10  "Object_Orientation"
  Bus Selector7/4 -> Data Type Conversion26/1  "<P0ArG>"
  HWA_Task100ms1/20(DesireDis) -> Bus Creator/20
  HWA_Task100ms1/3(P3ID) -> Bus Creator/3
  [ACCTargetSelectSts] -> Bus Selector7/1
  HWA_Task100ms1/27(ObjSpwRight) -> Bus Creator/27
  HWA_Task100ms1/18(CutIn_b) -> Bus Creator/18
  Bus Selector9/2 -> Data Type Conversion2/1  "<LH_Line_First_C1>"
  Data Type Conversion16/1 -> HWA_Task100ms1/18(VxvRef_ms)
  HWA_Task100ms1/35(bPC0) -> Bus Creator/35
  Bus Selector1/11 -> Selector9/1  "<ObjMoveSts>"
  HWA_Task100ms1/13(P2Dx) -> Bus Creator/13
  HWA_Task100ms1/30(ObjPlausRight) -> Bus Creator/30
  Bus Selector8/3 -> Data Type Conversion50/1  "<TarLineC1>"
  HWA_Task100ms1/16(P2Dy) -> Bus Creator/16
  HWA_Task100ms1/24(ObjVyc_ms) -> Bus Creator/24
  HWA_Task100ms1/21(Signal_ACC_TgtObjBarDisp) -> Bus Creator/21
  Data Type Conversion39/1 -> Bus Creator1/17  "P0HeadingAngle"
  HWA_Task100ms1/33(dxC0) -> Bus Creator/33
  HWA_Task100ms1/15(P0Dy) -> Bus Creator/15
  Data Type Conversion14/1 -> HWA_Task100ms1/16(TimeGap)
  HWA_Task100ms1/4(TargetBrake_b) -> Bus Creator/4
  Data Type Conversion47/1 -> HWA_Task100ms1/24(TarLineValid)
  Constant/1 -> Data Type Conversion35/1, Data Type Conversion34/1, Data Type Conversion31/1, Data Type Conversion30/1
  Bus Selector1/3 -> Selector3/1  "<ObjLatPos>"
  Bus Selector5/2 -> Data Type Conversion17/1  "<kapTraj>"
  Bus Selector7/5 -> Data Type Conversion27/1  "<P0Range>"
  Bus Selector1/5 -> Selector5/1  "<ObjClassification>"
  HWA_Task100ms1/31(ObjDycHist) -> Bus Creator/31
  Bus Creator/1 -> [ACCTargetSelectSts]
  Data Type Conversion21/1 -> HWA_Task100ms1/23(LongitudeAcc)
  Data Type Conversion23/1 -> Bus Creator1/2  "dxP0"
  TimeGap/1 -> Data Type Conversion14/1
  Data Type Conversion25/1 -> Bus Creator1/4  "ACCTgtObjVy"
  HWA_Task100ms1/11(P3ArG) -> Bus Creator/11
  Data Type Conversion30/1 -> Bus Creator1/9  "ObjMovingStateP0"
  Data Type Conversion18/1 -> HWA_Task100ms1/20(AlpSideSlipAngle)
  HWA_Task100ms1/22(ObjDyc_m) -> Bus Creator/22
  ACCMode/1 -> Data Type Conversion15/1
  Data Type Conversion49/1 -> HWA_Task100ms1/25(TarLine_A2)
  Bus Selector1/8 -> Selector8/1  "<ObjLongAccel>"
  HWA_Task100ms1/8(P3Vr) -> Bus Creator/8
  Bus Selector1/7 -> Selector7/1  "<ObjLatVel>"
  Data Type Conversion28/1 -> Bus Creator1/7  "targetExistP0"
  Data Type Conversion17/1 -> HWA_Task100ms1/19(kapCurvTraj)
  Bus Selector5/1 -> Data Type Conversion16/1  "<vxvRefMs>"
  Bus Selector8/1 -> Data Type Conversion47/1  "<TarLineValid>"
  Data Type Conversion34/1 -> Bus Creator1/13  "ACCTgtObjObstcl"
  VCAN/1 -> Bus Selector3/1
  Data Type Conversion35/1 -> Bus Creator1/14  "ACCTgtObjAy"
  Data Type Conversion32/1 -> Bus Creator1/11  "ObjTypeP0"
  HWA_Task100ms1/32(ObjqDycHist) -> Bus Creator/32
  Bus Selector7/8 -> Data Type Conversion40/1  "<TargetCutIn_b>"
  Data Type Conversion29/1 -> Bus Creator1/8  "fu_typeP0"
  Bus Selector7/2 -> Data Type Conversion23/1  "<P0Dx>"
  Bus Selector7/6 -> Data Type Conversion33/1  "<P0Dy>"
  Data Type Conversion38/1 -> Bus Creator1/16  "ACCTgtObjExist"
  VIE/1 -> Bus Selector5/1
  Bus Selector9/1 -> Data Type Conversion1/1  "<LH_Line_First_C2>"
  Bus Selector7/3 -> Data Type Conversion24/1  "<P0Vr>"
  Data Type Conversion19/1 -> HWA_Task100ms1/21(AlpWheelAngle)
  Bus Selector1/9 -> Selector10/1  "<ObjWidth>"
  Bus Selector3/1 -> Data Type Conversion21/1  "<VehLgtAccel>"
  HWA_Task100ms1/1(P0ID) -> Bus Creator/1
  Data Type Conversion37/1 -> Bus Creator1/15  "ACCTgtObjCntAlive"
  Data Type Conversion2/1 -> HWA_Task100ms1/14(A1)
  HWA_Task100ms1/2(P2ID) -> Bus Creator/2
  Data Type Conversion1/1 -> HWA_Task100ms1/13(A2)
  Data Type Conversion27/1 -> Bus Creator1/6  "rangeP0"
  Data Type Conversion22/1 -> Bus Creator1/1  "IDP0"
  Data Type Conversion3/1 -> HWA_Task100ms1/15(Conf)
  Bus Selector7/1 -> Data Type Conversion22/1  "<P0ID>"
  HWA_Task100ms1/38(bPC1) -> Bus Creator/38
  HWA_Task100ms1/34(aPC0) -> Bus Creator/34
  FilterTime6/1 -> Sum4/2
  Constant11/1 -> FilterTime3/3
  Sum4/1 -> FilterTime3/1
  FilterTime3/1 -> [alpWheelAngle]
  Bus Selector5/5 -> Sum4/1  "<SteerAngleOffset_deg>"
  Constant9/1 -> FilterTime3/2
  VCAN1/1 -> Bus Selector2/1
  Constant10/1 -> Sum1/2
  Gain9/1 -> FilterTime6/1
  Sum1/1 -> Gain9/1
  Bus Selector2/1 -> Data Type Conversion4/1  "<SteerWheelAngSign>"
  Bus Selector2/2 -> FilterTime6/2  "<SteerWheelAng>"
  Data Type Conversion4/1 -> Sum1/1
  HWA_Task100ms1/44(dOTL) -> Data Type Conversion10/1  "OTL_C0"
  HWA_Task100ms1/45(dxMaxOTL) -> Data Type Conversion11/1  "OTL_Range"
  rollingcounter 1/1(cnt) -> Data Type Conversion37/1, Data Type Conversion5/1  "OTL_Cnt"
  HWA_Task100ms1/43(cOTL) -> Data Type Conversion9/1  "OTL_C1"
  HWA_Task100ms1/40(OTLValid) -> Data Type Conversion6/1  "OTL_Valid"
  HWA_Task100ms1/41(aOTL) -> Data Type Conversion7/1  "OTL_C3"
  HWA_Task100ms1/42(bOTL) -> Data Type Conversion8/1  "OTL_C2"
  Bus Creator2/1 -> TEM_P0_TARGET_LINE/1
  Data Type Conversion5/1 -> Bus Creator2/7  "OTL_Cnt"
  Data Type Conversion6/1 -> Bus Creator2/1  "OTL_Valid"
  Data Type Conversion7/1 -> Bus Creator2/2  "OTL_C3"
  Data Type Conversion8/1 -> Bus Creator2/3  "OTL_C2"
  Data Type Conversion9/1 -> Bus Creator2/4  "OTL_C1"
  Data Type Conversion10/1 -> Bus Creator2/5  "OTL_C0"
  Data Type Conversion11/1 -> Bus Creator2/6  "OTL_Range"
  visMsg/1 -> Bus Selector/1
  Bus Selector/2 -> Selector/1  "<EQ4_LH_ELEM>"
  Selector/1 -> Bus Selector9/1
  Selector1/1 -> HWA_Task100ms1/1(ObjRange_m)
  Bias/1 -> HWA_Task100ms1/2(ObjDx_m)
  Selector3/1 -> HWA_Task100ms1/3(ObjDy_m)
  Selector4/1 -> HWA_Task100ms1/4(ObjValid)
  Selector5/1 -> HWA_Task100ms1/5(ObjClassification)
  Selector6/1 -> HWA_Task100ms1/6(ObjVxG_ms)
  Selector7/1 -> HWA_Task100ms1/7(ObjVyG_ms)
  Selector8/1 -> HWA_Task100ms1/8(ObjArG_ms2)
  Selector9/1 -> HWA_Task100ms1/11(ObjMoveSts)
  Selector10/1 -> HWA_Task100ms1/9(ObjWidth_m)
  Selector11/1 -> HWA_Task100ms1/12(ObjBrakeLightIndic)
  Selector12/1 -> HWA_Task100ms1/10(ObjCnt)
  Bus Selector/1 -> ObjMatrixTransit/1(EQ4_OBJ)  "<EQ4_OBJ>"
  ObjMatrixTransit/1(VisObjSts) -> Bus Selector1/1
  [ACCTargetSelectSts] -> Bus Selector4/1
  Bus Selector4/1 -> Compare To Constant/1, Data Type Conversion/1  "<P2ID>"
  Data Type Conversion/1 -> Bus Creator3/1  "IDP2"
  Bus Selector4/2 -> Data Type Conversion12/1  "<P2Dx>"
  Data Type Conversion12/1 -> Add/1, Bus Creator3/2  "dxP2"
  Bus Selector4/3 -> Data Type Conversion13/1  "<P2Vr>"
  Data Type Conversion13/1 -> Bus Creator3/3  "vxRelP2"
  Bus Selector4/4 -> Data Type Conversion36/1  "<P2ArG>"
  Data Type Conversion36/1 -> Bus Creator3/4  "axAbsGroundP2"
  Add/1 -> Bus Creator3/5  "rangeP2"
  Constant1/1 -> Add/2
  Compare To Constant/1 -> Bus Creator3/6  "targetExistP2"
  Constant2/1 -> Bus Creator3/7  "fu_typeP2"
  Constant3/1 -> Bus Creator3/8  "ObjMovingStateP2"
  Constant4/1 -> Bus Creator3/9  "ObjTypeP2"
  Bus Selector4/5 -> Data Type Conversion41/1  "<P2Dy>"
  Data Type Conversion41/1 -> Bus Creator3/10  "ObjDYP2"
  Constant5/1 -> Bus Creator3/11  "P2CutinProb"
  Constant6/1 -> Bus Creator3/12  "P2HeadingAngle"
  Bus Creator3/1 -> ACCP2/1
  Bus Creator4/1 -> ACCP3/1
  Constant15/1 -> Bus Creator4/12  "P3HeadingAngle"
  Constant14/1 -> Bus Creator4/11  "P3CutinProb"
  Data Type Conversion48/1 -> Bus Creator4/10  "ObjDYP3"
  Bus Selector6/5 -> Data Type Conversion48/1  "<P3Dy>"
  Constant13/1 -> Bus Creator4/9  "ObjTypeP3"
  Constant12/1 -> Bus Creator4/8  "ObjMovingStateP3"
  Constant8/1 -> Bus Creator4/7  "fu_typeP3"
  Compare To Constant1/1 -> Bus Creator4/6  "targetExistP3"
  Constant7/1 -> Add1/2
  Add1/1 -> Bus Creator4/5  "rangeP3"
  Data Type Conversion45/1 -> Bus Creator4/4  "axAbsGroundP3"
  Bus Selector6/4 -> Data Type Conversion45/1  "<P3ArG>"
  Data Type Conversion44/1 -> Bus Creator4/3  "vxRelP3"
  Bus Selector6/3 -> Data Type Conversion44/1  "<P3Vr>"
  Data Type Conversion43/1 -> Bus Creator4/2, Add1/1  "dxP3"
  Bus Selector6/2 -> Data Type Conversion43/1  "<P3Dx>"
  Data Type Conversion42/1 -> Bus Creator4/1  "IDP3"
  Bus Selector6/1 -> Data Type Conversion42/1, Compare To Constant1/1  "<P3ID>"
  [ACCTargetSelectSts] -> Bus Selector6/1
  Selector2/1 -> Bias/1
  Constant16/1 -> Data Type Conversion29/1
  Constant17/1 -> Data Type Conversion32/1
  HWA_Task100ms1/46(TargetVyG) -> Data Type Conversion25/1
  Constant18/1 -> Data Type Conversion39/1
  Data Type Conversion46/1 -> Terminator/1
  Data Type Conversion51/1 -> HWA_Task100ms1/27(TarLine_A0)

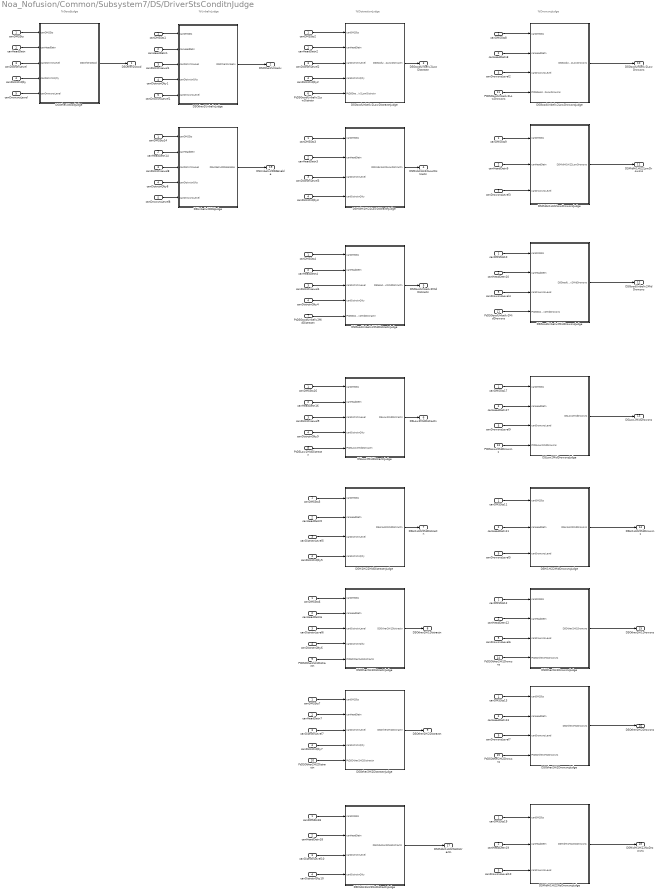
== system Noa_Nofusion/Common/Subsystem7/DS/DriverStsConditnJudge ==
  note: %GoodJudge
  note: %UnbelivJudge
  note: %DistractionJudge
  note: %DrowsnsJudge
  canDMSSts : Inport
  canHeadDetn : Inport  Port=2
  canDistrctnLevel : Inport  Port=3
  canDistrctnQlty : Inport  Port=4
  canDrowsnsLevel : Inport  Port=5
  PtDSGoodUnbeliv2LowDistrctn : Inport  Port=6
  PtDSGoodUnbeliv2MidDistractn : Inport  Port=7
  PtDSLow2MidDistractn : Inport  Port=8
  PtDSOther2Hi1Distractn : Inport  Port=9
  PtDSOther2Hi2Distractn : Inport  Port=10
  PtDSGoodUnbeliv2LowDrowsns : Inport  Port=11
  PtDSGoodUnbeliv2MidDrowsns : Inport  Port=12
  PtDSLow2MidDrowsns : Inport  Port=13
  PtDSOther2Hi1Drowsns : Inport  Port=14
  PtDSOther2Hi2Drowsns : Inport  Port=15
  DSGoodUnbeliv2LowDistractnJudge : Subsystem
  DSGoodUnbeliv2LowDrowsnsJudge : Subsystem
  DSGoodUnbeliv2MidDistractnJudge : Subsystem
  DSGoodUnbeliv2MidDrowsnsJudge : Subsystem
  DSHi1Hi22MidDistractnJudge : Subsystem
  DSHi1Hi22MidDrowsnsJudge : Subsystem
  DSLow2MidDistractnJudge : Subsystem
  DSLow2MidDrowsnsJudge : Subsystem
  DSMidHi1Hi22LowDistractnJudge : Subsystem
  DSMidHi1Hi22LowDrowsnsJudge : Subsystem
  DSMidHi1Hi22NoDistractnJudge : Subsystem
  DSMidHi1Hi22NoDrowsnsJudge : Subsystem
  DSOther2GoodJudge : Subsystem
  DSOther2Hi1DistractnJudge : Subsystem
  DSOther2Hi1DrowsnsJudge : Subsystem
  DSOther2Hi2DistractnJudge : Subsystem
  DSOther2Hi2DrowsnsJudge : Subsystem
  DSOther2UnbelivJudge : Subsystem
  DSUnbeliv2DDAJudge : Subsystem
  canDMSSts{1..14,16..19} (18 alike) : InportShadow
  canDistrctnLevel{1..10} (10 alike) : InportShadow  Port=3
  canDistrctnQlty{1..10} (10 alike) : InportShadow  Port=4
  canDrowsnsLevel{1..10} (10 alike) : InportShadow  Port=5
  canHeadDetn{1..14,16..19} (18 alike) : InportShadow  Port=2
  DSOther2Good : Outport
  DSOther2Unbeliv : Outport  Port=2
  DSGoodUnbeliv2LowDistractn : Outport  Port=3
  DSMidHi1Hi22LowDistractn : Outport  Port=4
  DSGoodUnbeliv2MidDistractn : Outport  Port=5
  DSLow2MidDistractn : Outport  Port=6
  DSHi1Hi22MidDistractn : Outport  Port=7
  DSOther2Hi1Distractn : Outport  Port=8
  DSOther2Hi2Distractn : Outport  Port=9
  DSGoodUnbeliv2LowDrowsns : Outport  Port=10
  DSMidHi1Hi22LowDrowsns : Outport  Port=11
  DSGoodUnbeliv2MidDrowsns : Outport  Port=12
  DSLow2MidDrowsns : Outport  Port=13
  DSHi1Hi22MidDrowsns : Outport  Port=14
  DSOther2Hi1Drowsns : Outport  Port=15
  DSOther2Hi2Drowsns : Outport  Port=16
  DSMidHi1Hi22NoDistractn : Outport  Port=17
  DSMidHi1Hi22NoDrowsns : Outport  Port=18
  DSUnbeliv2DDAEnable : Outport  Port=19
  wires:
  canDMSSts/1 -> DSOther2GoodJudge/1(canDMSSts)
  DSOther2GoodJudge/1(DSOther2Good) -> DSOther2Good/1
  canHeadDetn/1 -> DSOther2GoodJudge/2(canHeadDetn)
  canDistrctnLevel/1 -> DSOther2GoodJudge/3(canDistrctnLevel)
  canDistrctnQlty/1 -> DSOther2GoodJudge/4(canDistrctnQlty)
  canDrowsnsLevel/1 -> DSOther2GoodJudge/5(canDrowsnsLevel)
  canDMSSts1/1 -> DSOther2UnbelivJudge/1(canDMSSts)
  canHeadDetn1/1 -> DSOther2UnbelivJudge/2(canHeadDetn)
  canDistrctnLevel1/1 -> DSOther2UnbelivJudge/3(canDistrctnLevel)
  canDistrctnQlty1/1 -> DSOther2UnbelivJudge/4(canDistrctnQlty)
  canDrowsnsLevel1/1 -> DSOther2UnbelivJudge/5(canDrowsnsLevel)
  DSOther2UnbelivJudge/1(DSOther2Unbeliv) -> DSOther2Unbeliv/1
  DSGoodUnbeliv2LowDistractnJudge/1(DSGoodUnbeliv2LowDistractn) -> DSGoodUnbeliv2LowDistractn/1
  canDMSSts2/1 -> DSGoodUnbeliv2LowDistractnJudge/1(canDMSSts)
  canHeadDetn2/1 -> DSGoodUnbeliv2LowDistractnJudge/2(canHeadDetn)
  canDistrctnLevel2/1 -> DSGoodUnbeliv2LowDistractnJudge/3(canDistrctnLevel)
  canDistrctnQlty2/1 -> DSGoodUnbeliv2LowDistractnJudge/4(canDistrctnQlty)
  canDMSSts3/1 -> DSMidHi1Hi22LowDistractnJudge/1(canDMSSts)
  canHeadDetn3/1 -> DSMidHi1Hi22LowDistractnJudge/2(canHeadDetn)
  canDistrctnLevel3/1 -> DSMidHi1Hi22LowDistractnJudge/3(canDistrctnLevel)
  canDistrctnQlty3/1 -> DSMidHi1Hi22LowDistractnJudge/4(canDistrctnQlty)
  DSMidHi1Hi22LowDistractnJudge/1(DSMidHi1Hi22LowDistractn) -> DSMidHi1Hi22LowDistractn/1
  canDMSSts4/1 -> DSGoodUnbeliv2MidDistractnJudge/1(canDMSSts)
  canHeadDetn4/1 -> DSGoodUnbeliv2MidDistractnJudge/2(canHeadDetn)
  canDistrctnLevel4/1 -> DSGoodUnbeliv2MidDistractnJudge/3(canDistrctnLevel)
  canDistrctnQlty4/1 -> DSGoodUnbeliv2MidDistractnJudge/4(canDistrctnQlty)
  DSGoodUnbeliv2MidDistractnJudge/1(DSGoodUnbeliv2MidDistractn) -> DSGoodUnbeliv2MidDistractn/1
  canDMSSts5/1 -> DSHi1Hi22MidDistractnJudge/1(canDMSSts)
  canHeadDetn5/1 -> DSHi1Hi22MidDistractnJudge/2(canHeadDetn)
  canDistrctnLevel5/1 -> DSHi1Hi22MidDistractnJudge/3(canDistrctnLevel)
  canDistrctnQlty5/1 -> DSHi1Hi22MidDistractnJudge/4(canDistrctnQlty)
  DSHi1Hi22MidDistractnJudge/1(DSHi1Hi22MidDistractn) -> DSHi1Hi22MidDistractn/1
  DSOther2Hi1DistractnJudge/1(DSOther2Hi1Distractn) -> DSOther2Hi1Distractn/1
  canDMSSts6/1 -> DSOther2Hi1DistractnJudge/1(canDMSSts)
  canHeadDetn6/1 -> DSOther2Hi1DistractnJudge/2(canHeadDetn)
  canDistrctnLevel6/1 -> DSOther2Hi1DistractnJudge/3(canDistrctnLevel)
  canDistrctnQlty6/1 -> DSOther2Hi1DistractnJudge/4(canDistrctnQlty)
  DSOther2Hi2DistractnJudge/1(DSOther2Hi2Distractn) -> DSOther2Hi2Distractn/1
  canDMSSts7/1 -> DSOther2Hi2DistractnJudge/1(canDMSSts)
  canHeadDetn7/1 -> DSOther2Hi2DistractnJudge/2(canHeadDetn)
  canDistrctnLevel7/1 -> DSOther2Hi2DistractnJudge/3(canDistrctnLevel)
  canDistrctnQlty7/1 -> DSOther2Hi2DistractnJudge/4(canDistrctnQlty)
  DSGoodUnbeliv2LowDrowsnsJudge/1(DSGoodUnbeliv2LowDrowsns) -> DSGoodUnbeliv2LowDrowsns/1
  canDMSSts8/1 -> DSGoodUnbeliv2LowDrowsnsJudge/1(canDMSSts)
  canHeadDetn8/1 -> DSGoodUnbeliv2LowDrowsnsJudge/2(canHeadDetn)
  canDrowsnsLevel2/1 -> DSGoodUnbeliv2LowDrowsnsJudge/3(canDrowsnsLevel)
  DSMidHi1Hi22LowDrowsnsJudge/1(DSMidHi1Hi22LowDrowsns) -> DSMidHi1Hi22LowDrowsns/1
  canDMSSts9/1 -> DSMidHi1Hi22LowDrowsnsJudge/1(canDMSSts)
  canHeadDetn9/1 -> DSMidHi1Hi22LowDrowsnsJudge/2(canHeadDetn)
  canDrowsnsLevel3/1 -> DSMidHi1Hi22LowDrowsnsJudge/3(canDrowsnsLevel)
  canDMSSts10/1 -> DSGoodUnbeliv2MidDrowsnsJudge/1(canDMSSts)
  canHeadDetn10/1 -> DSGoodUnbeliv2MidDrowsnsJudge/2(canHeadDetn)
  canDrowsnsLevel4/1 -> DSGoodUnbeliv2MidDrowsnsJudge/3(canDrowsnsLevel)
  DSGoodUnbeliv2MidDrowsnsJudge/1(DSGoodUnbeliv2MidDrowsns) -> DSGoodUnbeliv2MidDrowsns/1
  DSHi1Hi22MidDrowsnsJudge/1(DSHi1Hi22MidDrowsns) -> DSHi1Hi22MidDrowsns/1
  canDrowsnsLevel5/1 -> DSHi1Hi22MidDrowsnsJudge/3(canDrowsnsLevel)
  canHeadDetn11/1 -> DSHi1Hi22MidDrowsnsJudge/2(canHeadDetn)
  canDMSSts11/1 -> DSHi1Hi22MidDrowsnsJudge/1(canDMSSts)
  canDMSSts12/1 -> DSOther2Hi1DrowsnsJudge/1(canDMSSts)
  canHeadDetn12/1 -> DSOther2Hi1DrowsnsJudge/2(canHeadDetn)
  canDrowsnsLevel6/1 -> DSOther2Hi1DrowsnsJudge/3(canDrowsnsLevel)
  DSOther2Hi1DrowsnsJudge/1(DSOther2Hi1Drowsns) -> DSOther2Hi1Drowsns/1
  canDrowsnsLevel7/1 -> DSOther2Hi2DrowsnsJudge/3(canDrowsnsLevel)
  canHeadDetn13/1 -> DSOther2Hi2DrowsnsJudge/2(canHeadDetn)
  canDMSSts13/1 -> DSOther2Hi2DrowsnsJudge/1(canDMSSts)
  DSOther2Hi2DrowsnsJudge/1(DSOther2Hi2Drowsns) -> DSOther2Hi2Drowsns/1
  DSLow2MidDistractnJudge/1(DSLow2MidDistractn) -> DSLow2MidDistractn/1
  canDistrctnQlty9/1 -> DSLow2MidDistractnJudge/4(canDistrctnQlty)
  canDistrctnLevel9/1 -> DSLow2MidDistractnJudge/3(canDistrctnLevel)
  canHeadDetn16/1 -> DSLow2MidDistractnJudge/2(canHeadDetn)
  canDMSSts16/1 -> DSLow2MidDistractnJudge/1(canDMSSts)
  canDrowsnsLevel9/1 -> DSLow2MidDrowsnsJudge/3(canDrowsnsLevel)
  canHeadDetn17/1 -> DSLow2MidDrowsnsJudge/2(canHeadDetn)
  canDMSSts17/1 -> DSLow2MidDrowsnsJudge/1(canDMSSts)
  DSLow2MidDrowsnsJudge/1(DSLow2MidDrowsns) -> DSLow2MidDrowsns/1
  canDistrctnQlty10/1 -> DSMidHi1Hi22NoDistractnJudge/4(canDistrctnQlty)
  canDistrctnLevel10/1 -> DSMidHi1Hi22NoDistractnJudge/3(canDistrctnLevel)
  canHeadDetn18/1 -> DSMidHi1Hi22NoDistractnJudge/2(canHeadDetn)
  canDMSSts18/1 -> DSMidHi1Hi22NoDistractnJudge/1(canDMSSts)
  DSMidHi1Hi22NoDistractnJudge/1(DSMidHi1Hi22NoDistractn) -> DSMidHi1Hi22NoDistractn/1
  canDrowsnsLevel10/1 -> DSMidHi1Hi22NoDrowsnsJudge/3(canDrowsnsLevel)
  canHeadDetn19/1 -> DSMidHi1Hi22NoDrowsnsJudge/2(canHeadDetn)
  canDMSSts19/1 -> DSMidHi1Hi22NoDrowsnsJudge/1(canDMSSts)
  DSMidHi1Hi22NoDrowsnsJudge/1(DSMidHi1Hi22NoDrowsns) -> DSMidHi1Hi22NoDrowsns/1
  canDrowsnsLevel8/1 -> DSUnbeliv2DDAJudge/5(canDrowsnsLevel)
  canDistrctnQlty8/1 -> DSUnbeliv2DDAJudge/4(canDistrctnQlty)
  canDistrctnLevel8/1 -> DSUnbeliv2DDAJudge/3(canDistrctnLevel)
  canHeadDetn14/1 -> DSUnbeliv2DDAJudge/2(canHeadDetn)
  canDMSSts14/1 -> DSUnbeliv2DDAJudge/1(canDMSSts)
  DSUnbeliv2DDAJudge/1(DSUnbeliv2DDAEnable) -> DSUnbeliv2DDAEnable/1
  PtDSGoodUnbeliv2LowDistrctn/1 -> DSGoodUnbeliv2LowDistractnJudge/5(PtDSGoodUnbeliv2LowDistrctn)
  PtDSGoodUnbeliv2MidDistractn/1 -> DSGoodUnbeliv2MidDistractnJudge/5(PtDSGoodUnbeliv2MidDistractn)
  PtDSLow2MidDistractn/1 -> DSLow2MidDistractnJudge/5(PtDSLow2MidDistractn)
  PtDSOther2Hi1Distractn/1 -> DSOther2Hi1DistractnJudge/5(PtDSOther2Hi1Distractn)
  PtDSOther2Hi2Distractn/1 -> DSOther2Hi2DistractnJudge/5(PtDSOther2Hi2Distractn)
  PtDSGoodUnbeliv2LowDrowsns/1 -> DSGoodUnbeliv2LowDrowsnsJudge/4(PtDSGoodUnbeliv2LowDrowsns)
  PtDSGoodUnbeliv2MidDrowsns/1 -> DSGoodUnbeliv2MidDrowsnsJudge/4(PtDSGoodUnbeliv2MidDrowsns)
  PtDSLow2MidDrowsns/1 -> DSLow2MidDrowsnsJudge/4(PtDSLow2MidDrowsns)
  PtDSOther2Hi1Drowsns/1 -> DSOther2Hi1DrowsnsJudge/4(PtDSOther2Hi1Drowsns)
  PtDSOther2Hi2Drowsns/1 -> DSOther2Hi2DrowsnsJudge/4(PtDSOther2Hi2Drowsns)
